simulink model "multiplemaximamodel2"  (R2023a)
settings: Solver=VariableStepAuto  StartTime=0.0  StopTime=10.0  RelTol=1e-3
libraries: spsPVArrayLib x15, spsDiodeLib x4, spsControlledVoltageSourceLib x2, spsCurrentMeasurementLib x2, simulink x2, spsVoltageMeasurementLib x2, sps_lib x1
settings Model: Creator=hp  LastModifiedBy=ask
settings SolverCC: AlgebraicLoopSolver=TrustRegion
settings DataIOCC: ReturnWorkspaceOutputs=off
settings DebuggingCC: UnconnectedInputMsg=warning  UnconnectedOutputMsg=warning  UnconnectedLineMsg=warning  ArithmeticOperatorsInVariantConditions=warning
settings ModelReferenceCC: EnableRefExpFcnMdlSchedulingChecks=on
settings SFSimCC: SimUseLocalCustomCode=off  CustomCodeUndefinedFunction=UseInterfaceOnly
settings RTWCC: RTWUseLocalCustomCode=off
settings CodeAppCC: StateflowObjectComments=on
settings SimscapeCC: SimscapeNormalizeSystem=off

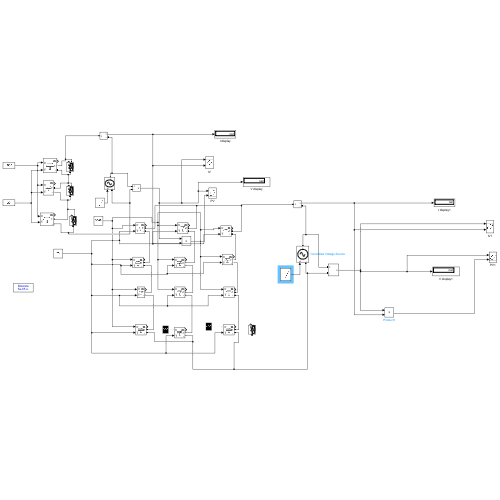
[thumbnail: Simulink's stored preview of the top-level diagram]
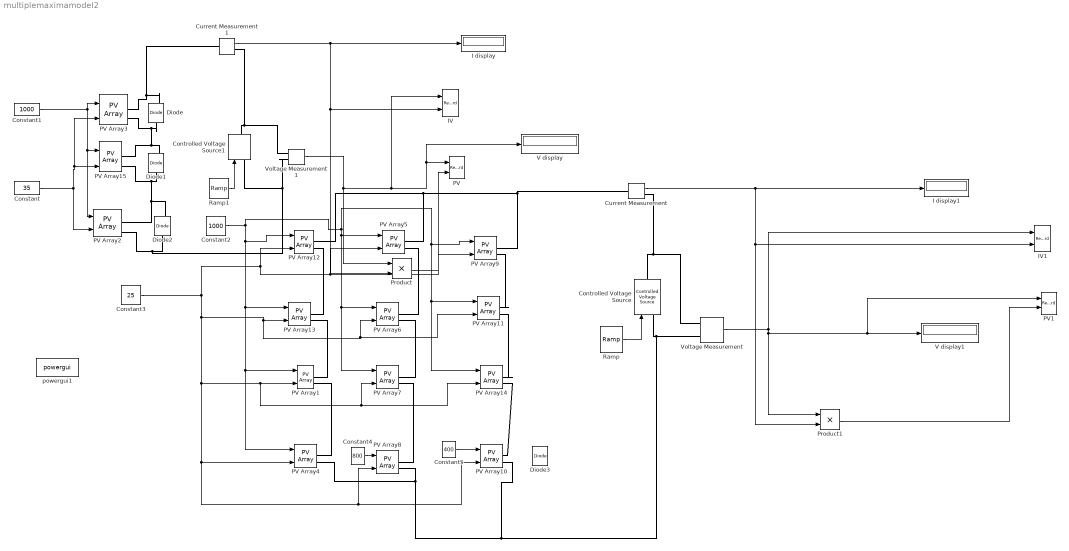
== system multiplemaximamodel2 ==
  Constant : Constant  Value=35
  Constant1 : Constant  Value=1000
  Constant2 : Constant  Value=1000
  Constant3 : Constant  Value=25
  Constant4 : Constant  Value=800
  Constant5 : Constant  Value=400
  Controlled Voltage Source : spsControlledVoltageSourceLib/Controlled Voltage Source  Initialize=on  Source_Type=AC  Amplitude=0  Phase=0  Frequency=0  Measurements=None
  Controlled Voltage Source1 : spsControlledVoltageSourceLib/Controlled Voltage Source  Initialize=on  Source_Type=AC  Amplitude=0  Phase=0  Frequency=0  Measurements=None
  Current Measurement : spsCurrentMeasurementLib/Current Measurement  PhasorSimulation=off  OutputType=Complex  PSBequivalent=0
  Current Measurement1 : spsCurrentMeasurementLib/Current Measurement  PhasorSimulation=off  OutputType=Complex  PSBequivalent=0
  Diode{,1..3} (4 alike) : spsDiodeLib/Diode  Ron=0.001  Lon=0  Vf=0.8  IC=0  UseSnubber=off  Rs=500  Cs=250e-9  Measurements=on
  I display : Display
  I display1 : Display
  IV : Record  FileSettingsInternal="{\"entries\":[{\"content\":{\"excelSettings\":{\"content\":{},\"type\":\"Streamout.ExcelSettings\"}},\"type\":\"Streamout.FileSettingStorage\",\"uuid\":\"34d25cae-9846-4861-85ea-62ad10805727\"}],\"packageUris\":[\"http://schema.mathworks.com/mf0/streamout_blocks/R2020a\"],\"version\":\"1.0\"}"  Layout=[1 1]  SignalsInternal="{\"entries\":[{\"content\":{\"signals\":[{\"content\":{\"blockPath\":[\"multiplemaximamodel2/IV\"],\"dimensions\":[1],\"domain\":\"multiplemaximamodel2/IV\",\"lineColor\":\"#a2142f\",\"plots\":[1],\"port\":1,\"sid\":[\"\"],\"signalID\":436,\"signalName\":\"Voltage Measurement1\"},\"type\":\"RecordBlkView.Signal\",\"uuid\":\"19c74cf0-de4f-4d0e-a147-9ff2f8316469\"},{\"content\":{\"blockPath\":[\"multiplemaximamodel2/IV\"],\"dimensions\":[1],\"domain\":\"multiplemaximamodel2/IV\",\"lineColor\":\"#139fff\",\"plots\":[1],\"port\":2,\"sid\":[\"\"],\"signalID\":440,\"signalName\":\"Current Measurement1\"},\"type\":\"RecordBlkView.Signal\",\"uuid\":\"be5394d9-6924-4bce-a224-b68786fce636\"}]},\"type\":\"RecordBlkView.InputSignals\",\"uuid\":\"d591409c-9ddf-4f69-80cd-c2a96de51d37\"}],\"packageUris\":[\"http://schema.mathworks.com/mf0/streamout_blocks/R2020a\"],\"version\":\"1.0\"}"  VisualizationBindings="{\"xyplotplugin\":{\"info\":[{\"series\":[{\"bindingParametersList\":[{\"parameter\":\"X-Axis\",\"signalID\":436,\"signalName\":\"Voltage Measurement1\"},{\"parameter\":\"Y-Axis\",\"signalID\":440,\"signalName\":\"Current Measurement1\"}],\"seriesID\":31342}],\"subplotID\":1}]}}"  CompatibilityTag=XY  st=-1
  IV1 : Record  FileSettingsInternal="{\"entries\":[{\"content\":{\"excelSettings\":{\"content\":{},\"type\":\"Streamout.ExcelSettings\"}},\"type\":\"Streamout.FileSettingStorage\",\"uuid\":\"e92ae03f-ef1e-4487-9559-32198ff1fc6d\"}],\"packageUris\":[\"http://schema.mathworks.com/mf0/streamout_blocks/R2020a\"],\"version\":\"1.0\"}"  Layout=[1 1]  SignalsInternal="{\"entries\":[{\"content\":{\"signals\":[{\"content\":{\"blockPath\":[\"multiplemaximamodel2/IV1\"],\"dimensions\":[1],\"domain\":\"multiplemaximamodel2/IV1\",\"lineColor\":\"#a2142f\",\"plots\":[1],\"port\":1,\"sid\":[\"\"],\"signalID\":420,\"signalName\":\"Voltage Measurement\"},\"type\":\"RecordBlkView.Signal\",\"uuid\":\"3b37f5b0-18fc-4226-b471-ab021e7d7752\"},{\"content\":{\"blockPath\":[\"multiplemaximamodel2/IV1\"],\"dimensions\":[1],\"domain\":\"multiplemaximamodel2/IV1\",\"lineColor\":\"#139fff\",\"plots\":[1],\"port\":2,\"sid\":[\"\"],\"signalID\":424,\"signalName\":\"Current Measurement\"},\"type\":\"RecordBlkView.Signal\",\"uuid\":\"cd9a5247-a523-4078-9d6e-1a413f04926d\"}]},\"type\":\"RecordBlkView.InputSignals\",\"uuid\":\"02668225-dd0c-42cb-b976-33b294020f8a\"}],\"packageUris\":[\"http://schema.mathworks.com/mf0/streamout_blocks/R2020a\"],\"version\":\"1.0\"}"  VisualizationBindings="{\"xyplotplugin\":{\"info\":[{\"series\":[{\"bindingParametersList\":[{\"parameter\":\"X-Axis\",\"signalID\":420,\"signalName\":\"Voltage Measurement\"},{\"parameter\":\"Y-Axis\",\"signalID\":424,\"signalName\":\"Current Measurement\"}],\"seriesID\":22192}],\"subplotID\":1}]}}"  CompatibilityTag=XY  st=-1
  PV : Record  FileSettingsInternal="{\"entries\":[{\"content\":{\"excelSettings\":{\"content\":{},\"type\":\"Streamout.ExcelSettings\"}},\"type\":\"Streamout.FileSettingStorage\",\"uuid\":\"f24bb543-d5b1-4655-8480-8cfb3e1afb4f\"}],\"packageUris\":[\"http://schema.mathworks.com/mf0/streamout_blocks/R2020a\"],\"version\":\"1.0\"}"  Layout=[1 1]  SignalsInternal="{\"entries\":[{\"content\":{\"signals\":[{\"content\":{\"blockPath\":[\"multiplemaximamodel2/PV\"],\"dimensions\":[1],\"domain\":\"multiplemaximamodel2/PV\",\"lineColor\":\"#a2142f\",\"plots\":[1],\"port\":1,\"sid\":[\"\"],\"signalID\":444,\"signalName\":\"Voltage Measurement1\"},\"type\":\"RecordBlkView.Signal\",\"uuid\":\"88418d48-7d49-48e1-8d75-afc81e9cc5dd\"},{\"content\":{\"blockPath\":[\"multiplemaximamodel2/PV\"],\"dimensions\":[1],\"domain\":\"multiplemaximamodel2/PV\",\"lineColor\":\"#139fff\",\"plots\":[1],\"port\":2,\"sid\":[\"\"],\"signalID\":448,\"signalName\":\"Product\"},\"type\":\"RecordBlkView.Signal\",\"uuid\":\"ffa5116a-533c-477a-a77e-122269fd28ce\"}]},\"type\":\"RecordBlkView.InputSignals\",\"uuid\":\"68ee7717-0ab0-46b3-ab99-b54abf64d913\"}],\"packageUris\":[\"http://schema.mathworks.com/mf0/streamout_blocks/R2020a\"],\"version\":\"1.0\"}"  VisualizationBindings="{\"xyplotplugin\":{\"info\":[{\"series\":[{\"bindingParametersList\":[{\"parameter\":\"X-Axis\",\"signalID\":444,\"signalName\":\"Voltage Measurement1\"},{\"parameter\":\"Y-Axis\",\"signalID\":448,\"signalName\":\"Product\"}],\"seriesID\":17417}],\"subplotID\":1}]}}"  CompatibilityTag=XY  st=-1
  PV Array{1..15} (15 alike) : spsPVArrayLib/PV Array  Npar=1  Nser=1  PlotType=array @ 1000 W/m2 & specified temperatures  S_vec="[ 1000  500  100 ]"  Temp_C_vec="[ 45 25  ]"  ModuleName=User-defined  PlotWhenSelected=off  Pm=213.15  Ncell=60  Voc=36.3  Isc=7.84  Vm=29  Im=7.35  beta_Voc_pc=-0.36099  alpha_Isc_pc=0.102  beta_Voc=-0.13104  alpha_Isc=0.0079968  IL=7.8654  I0=2.9273e-10  nI=0.98119  Rsh=313.0553  Rs=0.39381  RobustModel=off  RobustCellTemperature=313.3991  BAL=on  Tc=1e-6  Tfilter=5e-5
  PV1 : Record  FileSettingsInternal="{\"entries\":[{\"content\":{\"excelSettings\":{\"content\":{},\"type\":\"Streamout.ExcelSettings\"}},\"type\":\"Streamout.FileSettingStorage\",\"uuid\":\"20e93244-c43b-4bd4-9a7c-55f37539f328\"}],\"packageUris\":[\"http://schema.mathworks.com/mf0/streamout_blocks/R2020a\"],\"version\":\"1.0\"}"  Layout=[1 1]  SignalsInternal="{\"entries\":[{\"content\":{\"signals\":[{\"content\":{\"blockPath\":[\"multiplemaximamodel2/PV1\"],\"dimensions\":[1],\"domain\":\"multiplemaximamodel2/PV1\",\"lineColor\":\"#a2142f\",\"plots\":[1],\"port\":1,\"sid\":[\"\"],\"signalID\":428,\"signalName\":\"Voltage Measurement\"},\"type\":\"RecordBlkView.Signal\",\"uuid\":\"546c0ccb-926e-41fb-b502-2fe2248c19b8\"},{\"content\":{\"blockPath\":[\"multiplemaximamodel2/PV1\"],\"dimensions\":[1],\"domain\":\"multiplemaximamodel2/PV1\",\"lineColor\":\"#139fff\",\"plots\":[1],\"port\":2,\"sid\":[\"\"],\"signalID\":432,\"signalName\":\"Product1\"},\"type\":\"RecordBlkView.Signal\",\"uuid\":\"9802eb96-e946-4a16-bf19-c8d49cfd475a\"}]},\"type\":\"RecordBlkView.InputSignals\",\"uuid\":\"74c69acb-9603-4fa2-924f-b183c0c0efd0\"}],\"packageUris\":[\"http://schema.mathworks.com/mf0/streamout_blocks/R2020a\"],\"version\":\"1.0\"}"  VisualizationBindings="{\"xyplotplugin\":{\"info\":[{\"series\":[{\"bindingParametersList\":[{\"parameter\":\"X-Axis\",\"signalID\":428,\"signalName\":\"Voltage Measurement\"},{\"parameter\":\"Y-Axis\",\"signalID\":432,\"signalName\":\"Product1\"}],\"seriesID\":19120}],\"subplotID\":1}]}}"  CompatibilityTag=XY  st=-1
  Product : Product
  Product1 : Product
  Ramp : simulink/Sources/Ramp  slope=145.2  start=0  InitialOutput=0
  Ramp1 : simulink/Sources/Ramp  slope=145.2  start=0  InitialOutput=0
  V display : Display
  V display1 : Display
  Voltage Measurement : spsVoltageMeasurementLib/Voltage Measurement  PhasorSimulation=off  OutputType=Complex  PSBequivalent=0
  Voltage Measurement1 : spsVoltageMeasurementLib/Voltage Measurement  PhasorSimulation=off  OutputType=Complex  PSBequivalent=0
  powergui1 : sps_lib/powergui  Priority=1  SimulationMode=Discrete  SampleTime=50e-6  frequency=60  Iterations=50  frequencyindice=0  Pbase=100e6  ErrMax=1e-4  UnitsV=kV  UnitsW=MW  buscounter=0  FunctionMessages=off  echomessages=off  EnableUseOfTLC=off  CurrentSourceSwitches=off  DisableSnubberDevices=off  DisableRonSwitches=off  DisableVfSwitches=off  DisplayEquations=off  AutomaticDiscreteSolvers=off  SolverType=Tustin/Backward Euler (TBE)  Interpol=off  ExternalGateDelay=off  methode=off  Ts=10  x0status=blocks  SPID=off  SwTol=0  HookPort=off  NonlinearTolerance=1e-4  nMaxIteration=100  ContinueOnMaxIteration=off  RestoreLinks=warning  ResistiveCurrentMeasurement=off  Frange=[0:2:500]  Ylog=off  Xlog=on  ShowGrid=off  save=off  variable=ZData  structure=0  ZoomFFT=off  StartTime=0.0  cycles=1  DisplayStyle=1  fundamental=60  FreqAxis=off  MaxFrequency=1000  frequencyindicesteady=1  RmsSteady=1  display=off
  wires:
  Constant1/1 -> PV Array3/1, PV Array2/1, PV Array15/1
  Constant/1 -> PV Array2/2, PV Array3/2, PV Array15/2
  Ramp1/1 -> Controlled Voltage Source1/1
  Current Measurement1/1 -> Product/2, IV/2, I display/1
  Product/1 -> PV/2
  Voltage Measurement1/1 -> IV/1, V display/1, PV/1, Product/1
  Constant5/1 -> PV Array10/1
  Current Measurement/1 -> Product1/2, IV1/2, I display1/1
  Product1/1 -> PV1/2
  Voltage Measurement/1 -> PV1/1, V display1/1, Product1/1, IV1/1
  Constant3/1 -> PV Array12/2, PV Array9/2, PV Array5/2, PV Array13/2, PV Array11/2, PV Array6/2, PV Array14/2, PV Array7/2, PV Array1/2, PV Array10/2, PV Array8/2, PV Array4/2
  Ramp/1 -> Controlled Voltage Source/1
  Constant2/1 -> PV Array7/1, PV Array6/1, PV Array5/1, PV Array9/1, PV Array14/1, PV Array11/1, PV Array12/1, PV Array13/1, PV Array4/1, PV Array1/1
  Constant4/1 -> PV Array8/1
  connections:
  Diode/RConn1 -- PV Array3/RConn1 -- Current Measurement1/LConn1
  Diode/LConn1 -- PV Array3/RConn2 -- PV Array15/RConn1 -- Diode1/RConn1
  Voltage Measurement1/LConn2 -- PV Array2/RConn2 -- Diode2/LConn1 -- Controlled Voltage Source1/LConn1
  PV Array15/RConn2 -- Diode1/LConn1 -- PV Array2/RConn1 -- Diode2/RConn1
  Controlled Voltage Source1/RConn1 -- Current Measurement1/RConn1 -- Voltage Measurement1/LConn1
  Current Measurement/LConn1 -- PV Array9/RConn1 -- PV Array5/RConn1 -- PV Array12/RConn1
  PV Array4/RConn2 -- PV Array8/RConn2 -- PV Array10/RConn2 -- Controlled Voltage Source/LConn1 -- Voltage Measurement/LConn2
  Current Measurement/RConn1 -- Voltage Measurement/LConn1 -- Controlled Voltage Source/RConn1
  PV Array13/RConn2 -- PV Array1/RConn1
  PV Array14/RConn1 -- PV Array11/RConn2
  PV Array11/RConn1 -- PV Array9/RConn2
  PV Array1/RConn2 -- PV Array4/RConn1
  PV Array7/RConn2 -- PV Array8/RConn1
  PV Array7/RConn1 -- PV Array6/RConn2
  PV Array14/RConn2 -- PV Array10/RConn1
  PV Array6/RConn1 -- PV Array5/RConn2
  PV Array13/RConn1 -- PV Array12/RConn2
